simulink model "lab07"  (Simulink 7.1)
settings: Solver=ode45  StartTime=0.0  StopTime=10.0  RelTol=1e-3
values from neighbouring files (symbols this model uses):
  A =     [lab07.mat]
  B =     [lab07.mat]
  C =     [lab07.mat]
  D =     [lab07.mat]
settings Model: Creator=ALUNO  LastModifiedBy=ALUNO

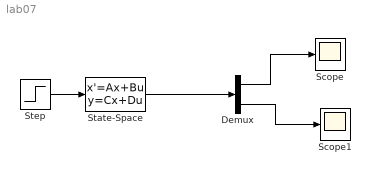
== system lab07 ==
  Demux : Demux  Outputs=[1 3]
  Scope : Scope
  Scope1 : Scope
  State-Space : StateSpace  A=A  B=B  C=C  D=D
  Step : Step  SampleTime=0
  wires:
  Step/1 -> State-Space/1
  Demux/1 -> Scope/1
  Demux/2 -> Scope1/1
  State-Space/1 -> Demux/1
